simulink model "buck_01_2018_b"  (Simulink 9.2)
settings: Solver=ode45  StartTime=0.0  StopTime=200/F  MaxStep=1/(10*F)  RelTol=1e-3  EnableMultiTasking=on
values from neighbouring files (symbols this model uses):
  C = 9.3e-6    (= 9.3e-06)    [buck_01_script.m]    (also in buck_02_script.m; buck_04_script.m)
  C1 = 5.5e-6    (= 5.5e-06)    [buck_01_script.m]    (also in buck_02_script.m; buck_04_script.m)
  duty = Vs / Ve    (= 0.66)    [buck_01_script.m]    (also in buck_02_script.m; buck_04_script.m)
  F = 500e3    (= 500000)    [buck_01_script.m]    (also in buck_02_script.m; buck_04_script.m)
  L = 1.9e-6    (= 1.9e-06)    [buck_01_script.m]    (also in buck_02_script.m; buck_04_script.m)
  L1 = 5e-6    (= 5e-06)    [buck_01_script.m]    (also in buck_02_script.m; buck_04_script.m)
  R = Vs^2 / Ps    (= 5.445)    [buck_01_script.m]    (also in buck_02_script.m = 0.5445; buck_04_script.m)
  Ve = 5    [buck_01_script.m]    (also in buck_02_script.m; buck_04_script.m)
libraries: powerlib x16
settings Model: Creator=lefrancp  LastModifiedBy=piffercg
settings DataIOCC: SignalLoggingSaveFormat=Dataset
settings DebuggingCC: UnderspecifiedInitializationDetection=Simplified  MergeDetectMultiDrivingBlocksExec=error  SolverPrmCheckMsg=warning  FcnCallInpInsideContextMsg=error  StateNameClashWarn=none
settings GRTTargetCC: GeneratePreprocessorConditionals=Use local settings  CombineOutputUpdateFcns=on  GRTInterface=off
settings ConfigComp: CovHtmlReporting=off  CovSFcnEnable=off
settings SimscapeCC: SimscapeNormalizeSystem=off

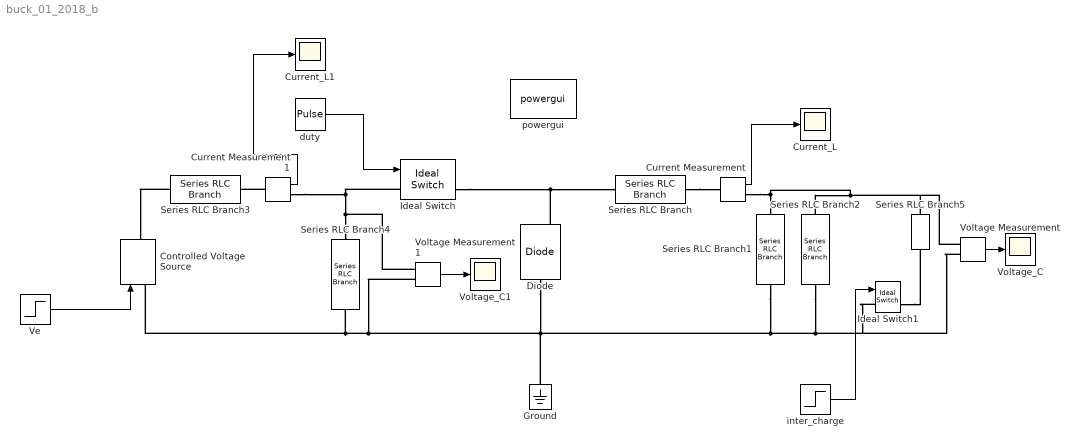
== system buck_01_2018_b ==
  Controlled Voltage Source : powerlib/Electrical Sources/Controlled Voltage Source  Initialize=on  Source_Type=AC  Amplitude=0  Phase=0  Frequency=0  Measurements=None
  Current Measurement : powerlib/Measurements/Current Measurement  PhasorSimulation=off  OutputType=Complex  PSBequivalent=0
  Current Measurement1 : powerlib/Measurements/Current Measurement  PhasorSimulation=off  OutputType=Complex  PSBequivalent=0
  Current_L : Scope
  Current_L1 : Scope
  Diode : powerlib/Power Electronics/Diode  Ron=0.001  Lon=0  Vf=0.01  IC=0  UseSnubber=off  Rs=500  Cs=250e-9  Measurements=on
  Ground : powerlib/Elements/Ground  LConnTagsString=a
  Ideal Switch : powerlib/Power Electronics/Ideal Switch  Ron=0.001  Lon=0  IC=0  Rs=1e5  Cs=inf  Measurements=on
  Ideal Switch1 : powerlib/Power Electronics/Ideal Switch  Ron=0.001  Lon=0  IC=0  Rs=1e5  Cs=inf  Measurements=on
  Series RLC Branch : powerlib/Elements/Series RLC Branch  LConnTagsString=__new0  RConnTagsString=__new0  BranchType=L  Resistance=1  Inductance=L  SetiL0=off  InitialCurrent=0  Capacitance=1e-6  Setx0=off  InitialVoltage=0  Measurements=None
  Series RLC Branch1 : powerlib/Elements/Series RLC Branch  LConnTagsString=__new0  RConnTagsString=__new0  BranchType=C  Resistance=1  Inductance=L  SetiL0=off  InitialCurrent=0  Capacitance=C  Setx0=off  InitialVoltage=0  Measurements=None
  Series RLC Branch2 : powerlib/Elements/Series RLC Branch  LConnTagsString=__new0  RConnTagsString=__new0  BranchType=R  Resistance=R  Inductance=L  SetiL0=off  InitialCurrent=0  Capacitance=C  Setx0=off  InitialVoltage=0  Measurements=None
  Series RLC Branch3 : powerlib/Elements/Series RLC Branch  LConnTagsString=__new0  RConnTagsString=__new0  BranchType=L  Resistance=1  Inductance=L1  SetiL0=off  InitialCurrent=0  Capacitance=1e-6  Setx0=off  InitialVoltage=0  Measurements=None
  Series RLC Branch4 : powerlib/Elements/Series RLC Branch  LConnTagsString=__new0  RConnTagsString=__new0  BranchType=C  Resistance=1  Inductance=L  SetiL0=off  InitialCurrent=0  Capacitance=C1  Setx0=off  InitialVoltage=0  Measurements=None
  Series RLC Branch5 : powerlib/Elements/Series RLC Branch  LConnTagsString=__new0  RConnTagsString=__new0  BranchType=R  Resistance=R*5  Inductance=L  SetiL0=off  InitialCurrent=0  Capacitance=C  Setx0=off  InitialVoltage=0  Measurements=None
  Ve : Step  Time=1e-4  Before=Ve  After=Ve+1  SampleTime=0
  Voltage Measurement : powerlib/Measurements/Voltage Measurement  PhasorSimulation=off  OutputType=Complex  PSBequivalent=0
  Voltage Measurement1 : powerlib/Measurements/Voltage Measurement  PhasorSimulation=off  OutputType=Complex  PSBequivalent=0
  Voltage_C : Scope
  Voltage_C1 : Scope
  duty : DiscretePulseGenerator  PulseType=Time based  Period=1/F  PulseWidth=duty*100
  inter_charge : Step  Time=2e-4  SampleTime=0
  powergui : powerlib/powergui  Priority=1  SimulationMode=Continuous  SampleTime=50e-6  frequency=60  Iterations=50  frequencyindice=0  Pbase=100e6  ErrMax=1e-4  UnitsV=kV  UnitsW=MW  buscounter=0  FunctionMessages=off  echomessages=off  EnableUseOfTLC=off  CurrentSourceSwitches=on  DisableSnubberDevices=off  DisableRonSwitches=off  DisableVfSwitches=off  DisplayEquations=off  SolverType=Tustin  Interpol=off  ExternalGateDelay=off  methode=off  Ts=0  x0status=blocks  SPID=off  SwTol=0  HookPort=off  RestoreLinks=warning  ResistiveCurrentMeasurement=off  Frange=[0:2:500]  Ylog=off  Xlog=on  ShowGrid=off  save=off  variable=ZData  structure=0  ZoomFFT=off  StartTime=0.0  cycles=1  DisplayStyle=1  fundamental=60  FreqAxis=off  MaxFrequency=1000  frequencyindicesteady=1  RmsSteady=1  display=off
  wires:
  Voltage Measurement/1 -> Voltage_C/1
  Current Measurement/1 -> Current_L/1
  duty/1 -> Ideal Switch/1
  Ve/1 -> Controlled Voltage Source/1
  Voltage Measurement1/1 -> Voltage_C1/1
  Current Measurement1/1 -> Current_L1/1
  inter_charge/1 -> Ideal Switch1/1
  connections:
  Series RLC Branch1/RConn1 -- Ideal Switch1/LConn1 -- Voltage Measurement/LConn2 -- Series RLC Branch2/RConn1 -- Voltage Measurement1/LConn2 -- Series RLC Branch4/RConn1 -- Controlled Voltage Source/LConn1 -- Ground/LConn1 -- Diode/LConn1
  Ideal Switch/RConn1 -- Diode/RConn1 -- Series RLC Branch/LConn1
  Series RLC Branch2/LConn1 -- Voltage Measurement/LConn1 -- Series RLC Branch5/LConn1 -- Current Measurement/RConn1 -- Series RLC Branch1/LConn1
  Series RLC Branch/RConn1 -- Current Measurement/LConn1
  Ideal Switch/LConn1 -- Current Measurement1/RConn1 -- Voltage Measurement1/LConn1 -- Series RLC Branch4/LConn1
  Series RLC Branch3/LConn1 -- Controlled Voltage Source/RConn1
  Current Measurement1/LConn1 -- Series RLC Branch3/RConn1
  Ideal Switch1/RConn1 -- Series RLC Branch5/RConn1
